simulink library "cec"  (Simulink 8.1)
settings: Solver=ode1  StartTime=0.0  StopTime=Inf  FixedStep=0.001  RelTol=1e-3
PostLoadFcn:
  | , if any(exist('dsrtsu_mdlpostloadfcn', 'file') == [2, 3, 6]), try dsrtsu_mdlpostloadfcn('Execute', bdroot); catch fprintf('Error in PostLoadFcn (dsrtsu_mdlpostloadfcn) for model "%s":\n %s\n', bdroot, lasterr); end, end,
undefined symbols (not defined in the file or in its folder): ENUM_KEYSWITCH_ON, ENUM_SENSORSTATE_NORMAL, FALSE, TRUE
settings Model: DSRTSU_INTERNAL_RTI_VER=450  DSRTSU_INTERNAL_RTI_TYPE=rti1401  RTICANMMDATA=struct('GeneralSetupData',struct('modelroot','D:\ELN150201_TAIWAN\trunk\AdasDragon\software\sw_development\arch\app\jud','generalsettings',struct('filesettings',struct('destfolder',struct('Name','RTICANMM_FILES','Check',1),'buildfolder',struct('Name','.','Check',1),'AbsDestfolder',struct('Name','D:\ELN150201_TAIWAN\trunk\AdasDragon\software\sw_development\arch\app\jud\RTICANMM_FILES'),'AbsBuildfolder',struct('Name','D:\ELN150201_TAIWAN\trunk\AdasDragon\software\sw_development\arch\app\jud'))),'options',struct('addpaths',1,'rmpaths',1,'addtrcexclusion',logical(1),'cannavigator',struct('checkmonitoring',0),'show_usrtrc',0,'use_usrtrc',0),'advanced',struct('options',[1 1 1 1 1 1 1 1 1 1 1 1 1 1 1 1 1 1 1 1 1 1 1 1 1 1 1 1 1 1 1 1 1 1 1 1 1 1 1 1 1 1 1 1 1 1 1 1 1 1 1 1 1 1 1 1 1 1 1 1 1 1 1 1 1 1 1 1 1 1 1 1 1 1 1 1 1 1 1 1 1 1 1 1 1 1 1 1 1 1 1 1 1 1 1 1 1 1 1 1]),'MPSetup',{{}},'modelname','cec','block','cec'))  DSRTSU_INTERNAL_RTIFPGA=40  Creator=AT015411  LastModifiedBy=AT015555

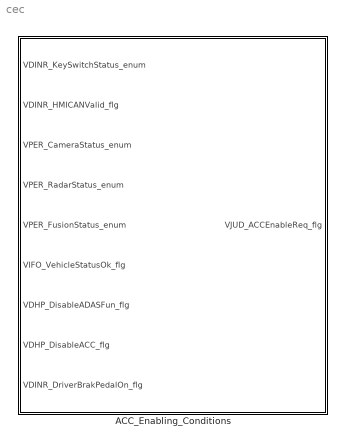
== system cec ==
  ACC_Enabling_Conditions : Subsystem

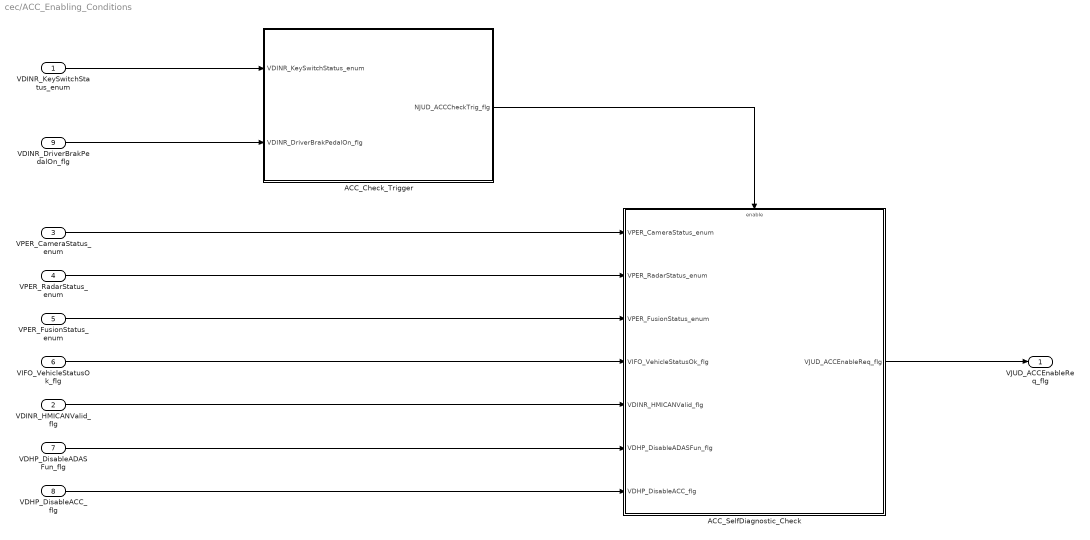
== system cec/ACC_Enabling_Conditions ==
  "VDINR_KeySwitchStatus_enum " : Inport
  VDINR_HMICANValid_flg : Inport  Port=2
  VPER_CameraStatus_enum : Inport  Port=3
  VPER_RadarStatus_enum : Inport  Port=4
  VPER_FusionStatus_enum : Inport  Port=5
  VIFO_VehicleStatusOk_flg : Inport  Port=6
  VDHP_DisableADASFun_flg : Inport  Port=7
  VDHP_DisableACC_flg : Inport  Port=8
  VDINR_DriverBrakPedalOn_flg : Inport  Port=9
  ACC_Check_Trigger : Subsystem
  ACC_SelfDiagnostic_Check : Subsystem
  VJUD_ACCEnableReq_flg : Outport
  wires:
  VDHP_DisableADASFun_flg/1 -> ACC_SelfDiagnostic_Check/6(VDHP_DisableADASFun_flg)
  VDHP_DisableACC_flg/1 -> ACC_SelfDiagnostic_Check/7(VDHP_DisableACC_flg)
  VDINR_HMICANValid_flg/1 -> ACC_SelfDiagnostic_Check/5(VDINR_HMICANValid_flg)
  VIFO_VehicleStatusOk_flg/1 -> ACC_SelfDiagnostic_Check/4(VIFO_VehicleStatusOk_flg)
  VPER_FusionStatus_enum/1 -> ACC_SelfDiagnostic_Check/3(VPER_FusionStatus_enum)
  VPER_RadarStatus_enum/1 -> ACC_SelfDiagnostic_Check/2(VPER_RadarStatus_enum)
  VPER_CameraStatus_enum/1 -> ACC_SelfDiagnostic_Check/1(VPER_CameraStatus_enum)
  ACC_SelfDiagnostic_Check/1(VJUD_ACCEnableReq_flg) -> VJUD_ACCEnableReq_flg/1
  "VDINR_KeySwitchStatus_enum "/1 -> ACC_Check_Trigger/1("VDINR_KeySwitchStatus_enum ")
  VDINR_DriverBrakPedalOn_flg/1 -> ACC_Check_Trigger/2(VDINR_DriverBrakPedalOn_flg)
  ACC_Check_Trigger/1(NJUD_ACCCheckTrig_flg) -> ACC_SelfDiagnostic_Check/Enable

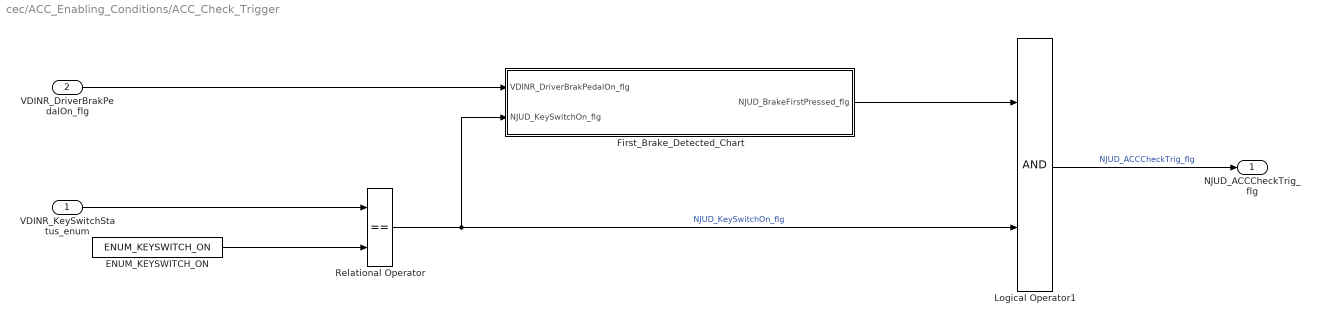
== system cec/ACC_Enabling_Conditions/ACC_Check_Trigger ==
  "VDINR_KeySwitchStatus_enum " : Inport
  VDINR_DriverBrakPedalOn_flg : Inport  Port=2
  ENUM_KEYSWITCH_ON : Constant  Value=ENUM_KEYSWITCH_ON  OutDataTypeStr=uint8
  First_Brake_Detected_Chart : Stateflow chart  TreatAsAtomicUnit=on
  Logical Operator1 : Logic  AllPortsSameDT=off  OutDataTypeStr=boolean
  Relational Operator : RelationalOperator  Operator===  OutDataTypeStr=boolean
  NJUD_ACCCheckTrig_flg : Outport
  wires:
  Logical Operator1/1 -> NJUD_ACCCheckTrig_flg/1  "NJUD_ACCCheckTrig_flg"
  "VDINR_KeySwitchStatus_enum "/1 -> Relational Operator/1
  ENUM_KEYSWITCH_ON/1 -> Relational Operator/2
  Relational Operator/1 -> First_Brake_Detected_Chart/2(NJUD_KeySwitchOn_flg), Logical Operator1/2  "NJUD_KeySwitchOn_flg"
  First_Brake_Detected_Chart/1(NJUD_BrakeFirstPressed_flg) -> Logical Operator1/1
  VDINR_DriverBrakPedalOn_flg/1 -> First_Brake_Detected_Chart/1(VDINR_DriverBrakPedalOn_flg)

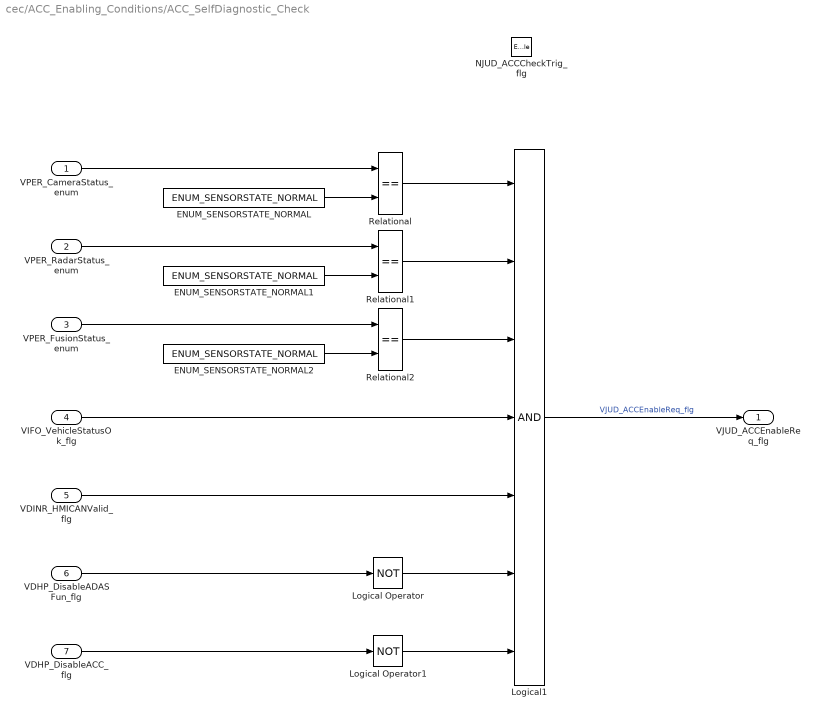
== system cec/ACC_Enabling_Conditions/ACC_SelfDiagnostic_Check ==
  VPER_CameraStatus_enum : Inport
  VPER_RadarStatus_enum : Inport  Port=2
  VPER_FusionStatus_enum : Inport  Port=3
  VIFO_VehicleStatusOk_flg : Inport  Port=4
  VDINR_HMICANValid_flg : Inport  Port=5
  VDHP_DisableADASFun_flg : Inport  Port=6
  VDHP_DisableACC_flg : Inport  Port=7
  NJUD_ACCCheckTrig_flg : EnablePort
      settings: AttributesFormatString=State = %<StatesWhenEnabling>
  ENUM_SENSORSTATE_NORMAL : Constant  Value=ENUM_SENSORSTATE_NORMAL  OutDataTypeStr=uint8
  ENUM_SENSORSTATE_NORMAL1 : Constant  Value=ENUM_SENSORSTATE_NORMAL  OutDataTypeStr=uint8
  ENUM_SENSORSTATE_NORMAL2 : Constant  Value=ENUM_SENSORSTATE_NORMAL  OutDataTypeStr=uint8
  Logical Operator : Logic  Operator=NOT  AllPortsSameDT=off  OutDataTypeStr=boolean
  Logical Operator1 : Logic  Operator=NOT  AllPortsSameDT=off  OutDataTypeStr=boolean
  Logical1 : Logic  Inputs=7  AllPortsSameDT=off  OutDataTypeStr=boolean
  Relational : RelationalOperator  Operator===  OutDataTypeStr=boolean
  Relational1 : RelationalOperator  Operator===  OutDataTypeStr=boolean
  Relational2 : RelationalOperator  Operator===  OutDataTypeStr=boolean
  VJUD_ACCEnableReq_flg : Outport  OutputWhenDisabled=reset  InitialOutput=0
  wires:
  VDHP_DisableACC_flg/1 -> Logical Operator1/1
  VDHP_DisableADASFun_flg/1 -> Logical Operator/1
  ENUM_SENSORSTATE_NORMAL2/1 -> Relational2/2
  VPER_FusionStatus_enum/1 -> Relational2/1
  ENUM_SENSORSTATE_NORMAL1/1 -> Relational1/2
  VPER_RadarStatus_enum/1 -> Relational1/1
  Logical1/1 -> VJUD_ACCEnableReq_flg/1  "VJUD_ACCEnableReq_flg"
  ENUM_SENSORSTATE_NORMAL/1 -> Relational/2
  VPER_CameraStatus_enum/1 -> Relational/1
  Relational/1 -> Logical1/1
  Relational1/1 -> Logical1/2
  Relational2/1 -> Logical1/3
  VIFO_VehicleStatusOk_flg/1 -> Logical1/4
  VDINR_HMICANValid_flg/1 -> Logical1/5
  Logical Operator/1 -> Logical1/6
  Logical Operator1/1 -> Logical1/7

== stateflow chart ACC_Enabling_Conditions/ACC_Check_Trigger/First_Brake_Detected_Chart ==
  state FIRST_PRESSED
    en:
    NJUD_BrakeFirstPressed_flg = TRUE;
  state INITIALIZATION
    en:
    NJUD_BrakeFirstPressed_flg = FALSE;
  (default) -> INITIALIZATION
  INITIALIZATION -> FIRST_PRESSED : [VDINR_DriverBrakPedalOn_flg==TRUE...
      | && NJUD_KeySwitchOn_flg==TRUE]
  FIRST_PRESSED -> INITIALIZATION : [NJUD_KeySwitchOn_flg==FALSE]
  data: NJUD_BrakeFirstPressed_flg output boolean =FALSE; TRUE parameter boolean; FALSE parameter boolean; VDINR_DriverBrakPedalOn_flg input double; NJUD_KeySwitchOn_flg input double
